simulink model "ElevatorControlSystem"  (R2024b)
settings: Solver=VariableStepAuto  StartTime=0.0  StopTime=inf  RelTol=1e-3
settings Model: Creator=rohan  LastModifiedBy=deepi

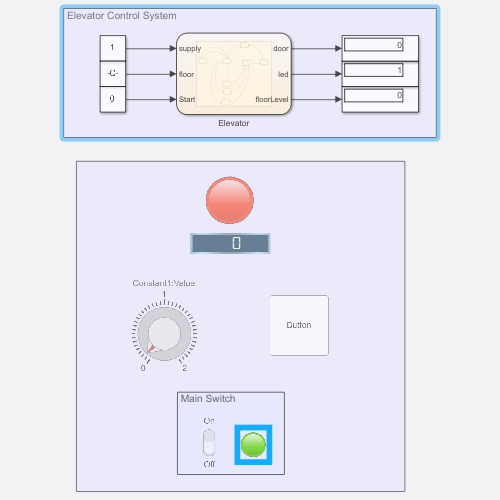
[thumbnail: Simulink's stored preview of the top-level diagram]
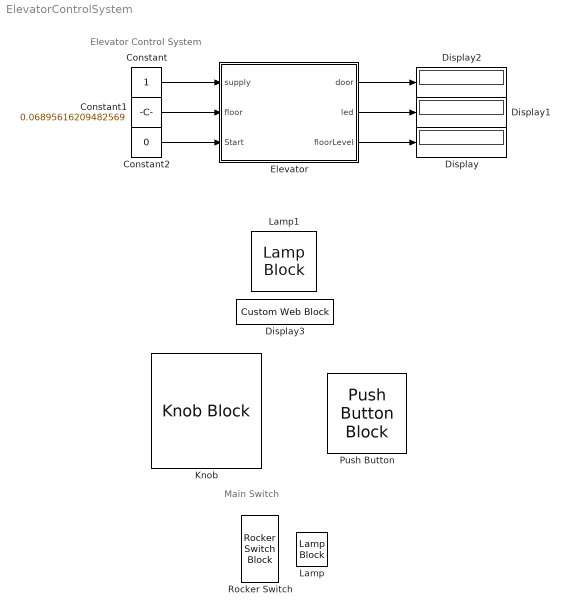
== system ElevatorControlSystem ==
  note: Main Switch
  note: Elevator Control System
  Constant : Constant
  Constant1 : Constant  Value=0.06895616209482569
  Constant2 : Constant  Value=0
  Display : Display
  Display1 : Display
  Display2 : Display
  Display3 : CustomWebBlock  LabelPosition=Hide  ShowInitialText=on  Configuration="{\"components\":[{\"name\":\"DisplayComponent\",\"settings\":{\"bold\":false,\"font\":\"DSEG7 Classic\",\"fontColor\":[255,255,200],\"fontSize\":\"14\",\"format\":\"short\",\"formatString\":\"%d\",\"italic\":false,\"position\":[0,0,1,1],\"underline\":false}},{\"name\":\"BackgroundImageComponent\",\"settings\":{\"image\":{\"size\":[300,80],\"src\":\"data:image\\/svg+xml;base64,PHN2ZyBpZD0iZnJhbWUiIHhtbG5zPSJodHRwOi8vd3d3LnczLm9yZy8yMDAwL3N2ZyIgeG1sbnM6eGxpbms9Imh0dHA6Ly93d3cudzMub3JnLzE5OTkveGxpbmsiIHZpZXdCb3g9IjAgMCAzODAgMTAxIj48ZGVmcz48c3R5bGU+LmNscy0xe2ZpbGw6IzAwMmI0Mjt9LmNscy0ye2ZpbGw6IzQyNzA4Mjt9LmNscy0ze2ZpbGw6dXJsKCNyYWRpYWwtZ3JhZGllbnQpO308L3N0eWxlPjxyYWRpYWxHcmFkaWVudCBpZD0icmFkaWFsLWdyYWRpZW50IiBjeD0iMTkwIiBjeT0iNTAuNSIgcj0iMjY5LjIxIiBncmFkaWVudFVuaXRzPSJ1c2VyU3BhY2VPblVzZSI+PHN0b3Agb2Zmc2V0PSIwLjAxIiBzdG9wLWNvbG9yPSIjM2U0ZjU4Ii8+PHN0b3Agb2Zmc2V0PSIwLjA2IiBzdG9wLWNvbG9yPSIjNDQ1NzYxIi8+PHN0b3Agb2Zmc2V0PSIwLjE1IiBzdG9wLWNvbG9yPSIjNTU2YTc2Ii8+PHN0b3Agb2Zmc2V0PSIwLjI1IiBzdG9wLWNvbG9yPSIjNmQ4ODk1Ii8+PHN0b3Agb2Zmc2V0PSIwLjM4IiBzdG9wLWNvbG9yPSIjOGZiMmMzIi8+PHN0b3Agb2Zmc2V0PSIwLjUyIiBzdG9wLWNvbG9yPSIjYjZlNGZhIi8+PHN0b3Agb2Zmc2V0PSIxIiBzdG9wLWNvbG9yPSIjMTU0NjU3Ii8+PC9yYWRpYWxHcmFkaWVudD48L2RlZnM+PGcgaWQ9IkxheWVyXzIiIGRhdGEtbmFtZT0iTGF5ZXIgMiI+PGcgaWQ9IkxheWVyXzEtMiIgZGF0YS1uYW1lPSJMYXllciAxLTIiPjxyZWN0IGlkPSJyZWN0MTAzNiIgY2xhc3M9ImNscy0xIiB4PSIxMSIgeT0iMTEiIHdpZHRoPSIzNTgiIGhlaWdodD0iNzkiLz48cGF0aCBpZD0icGF0aDEwMzgiIGNsYXNzPSJjbHMtMiIgZD0iTTgsOFY5M0gzNzJWOFpNMzY5LDkwSDExVjExSDM2OVoiLz48cGF0aCBpZD0icGF0aDEwNDAiIGNsYXNzPSJjbHMtMyIgZD0iTTAsMFYxMDFIMzgwVjBaTTM3Miw5M0g4VjhIMzcyWiIvPjwvZz48L2c+PC9zdmc+\",\"srcOrientation\":\"Right\"},\"position\":[0,0,1,1],\"scaleMode\":\"0\"}},{\"name\":\"ForegroundImageComponent\",\"settings\":{\"angle\":0,\"image\":{\"size\":[0,0],\"src\":\"default\"},\"isForeground\":1,\"position\":[0,0,1,1],\"scaleMode\":\"0\"}}],\"settings\":{\"BindingType\":\"signal\",\"aspectRatio\":1.032258064516129,\"backgroundColor\":[0,0,0,\"1\"],\"backgroundOffset\":0.14,\"backgroundOpacity\":1,\"fixedAspectRatio\":\"on\",\"showBackgroundColor\":false,\"value\":0,\"version\":\"R2023b\"},\"type\":\"Display\"}"
  Elevator : Stateflow chart  TreatAsAtomicUnit=on
  Knob : KnobBlock  ScaleMax=2  TickInterval=1
  Lamp : LampBlock  LabelPosition=Hide
  Lamp1 : LampBlock  LabelPosition=Hide
  Push Button : PushButtonBlock  OffValue=0.000000
  Rocker Switch : RockerSwitchBlock  LabelPosition=Hide
      settings: Values={{'Off', 'On'}, [0 1]}
  wires:
  Constant/1 -> Elevator/1(supply)
  Constant1/1 -> Elevator/2(floor)
  Elevator/3(floorLevel) -> Display/1
  Elevator/1(door) -> Display2/1
  Elevator/2(led) -> Display1/1
  Constant2/1 -> Elevator/3(Start)

== stateflow chart ElevatorControlSystem/Elevator ==
  state Elevator [group]
    state steady
      door==0
    state Power_supply1
      led=0
      door=5
    state floor_selector
      entry:
      led=1
      door=3
    state Door_close1
      door=0
    state Door_open1
      door=1
    state level_0
      floorLevel=0
    state level_1
      floorLevel=1
    state level_2
      floorLevel=2
    Door_close1 -> steady : after(2,sec)
    steady -> floor_selector : [Start==1]
    Power_supply1 -> floor_selector : [supply==1]
    floor_selector -> Power_supply1 [order 4] : [supply==0]
    (default) -> Power_supply1
    floor_selector -> level_2 [order 1] : [round(floor)==2&&...
        | supply==1]
    floor_selector -> level_1 [order 3] : [round(floor)==1 ...
        | &&supply==1]
    Door_open1 -> Door_close1 : after(5,sec)
    floor_selector -> level_0 [order 2] : [round(floor)==0 && ...
        | supply==1]
    level_2 -> Door_open1 : after(2,sec)
    level_0 -> Door_open1 : after(2,sec)
    level_1 -> Door_open1 : after(2,sec)
  data: supply input; door output; led output; floorLevel output; floor input; Start input
